simulink model "NN2_NetworkInverse"  (R2024b)
settings: Solver=FixedStepAuto  StartTime=0.0  StopTime=50  FixedStep=0.1  RelTol=1e-3
settings Model: Creator=azonh  LastModifiedBy=azonh

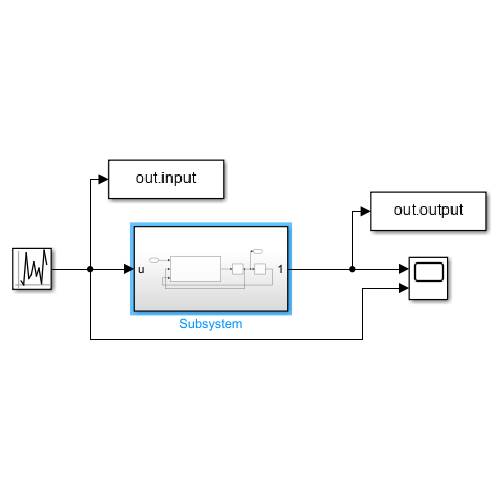
[thumbnail: Simulink's stored preview of the top-level diagram]
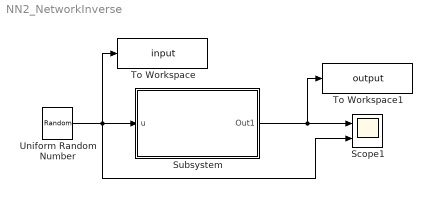
== system NN2_NetworkInverse ==
  Scope1 : Scope  NumInputPorts=2
  Subsystem : Subsystem
  To Workspace : ToWorkspace  VariableName=input  SampleTime=-1
  To Workspace1 : ToWorkspace  VariableName=output  SampleTime=-1
  Uniform Random Number : UniformRandomNumber  Minimum=-0.5  Maximum=0.5  SampleTime=0.1
  wires:
  Uniform Random Number/1 -> Scope1/2, To Workspace/1, Subsystem/1(u)
  Subsystem/1(Out1) -> Scope1/1, To Workspace1/1

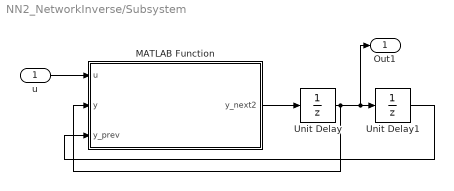
== system NN2_NetworkInverse/Subsystem ==
  u : Inport
  MATLAB Function : MATLAB Function  TreatAsAtomicUnit=on
  Unit Delay : UnitDelay  SampleTime=-1  HasFrameUpgradeWarning=on
  Unit Delay1 : UnitDelay  SampleTime=-1  HasFrameUpgradeWarning=on
  Out1 : Outport
  wires:
  u/1 -> MATLAB Function/1(u)
  Unit Delay/1 -> Out1/1, Unit Delay1/1, MATLAB Function/2(y)
  Unit Delay1/1 -> MATLAB Function/3(y_prev)
  MATLAB Function/1(y_next2) -> Unit Delay/1

== matlab function NN2_NetworkInverse/Subsystem/MATLAB Function ==
  data: u input; y input; y_next2 output; y_prev input
function y_next2 = fcn(u, y, y_prev)
    % u : commande actuelle u(t+1)
    % y : sortie actuelle y(t+1)
    % y_prev : sortie précédente y(t)
    
    % Équation non linéaire du document 
    y_next2 = 0.7653*y - 0.231*y_prev + ...
              0.4801*u - 0.6407*y^2 + ...
              1.014*y_prev*y - 0.3921*y^2 + ...
              0.592*y*u - 0.5611*y_prev*u;
end
